simulink model "acDynModelGolfTenueClassique"  (R2019a)
settings: Solver=VariableStepAuto  StartTime=0.0  StopTime=10  RelTol=1e-3
values from neighbouring files (symbols this model uses):
  DEG2RAD = pi/180.    (= 0.0174532925199)    [mainProjetCADV_2a.m]    (also in utAcDynamicsFunction.m; utConstantAeroCoeff.m)
  dPHRTrim = trimVal(1)    [mainProjetCADV_2a.m]
  dthrIdle = 0.1    [mainProjetCADV_2a.m]
  km = trim.kmass(choix)    [utGetTrimPoint.m]
  ms = trim.mStat(choix)    [utGetTrimPoint.m]
  RAD2DEG = 180/pi    (= 57.2957795131)    [mainProjetCADV_2a.m]    (also in utAcDynamicsFunction.m)
  thetaTrim = trimVal(3)    [mainProjetCADV_2a.m]
  xTrim = zeros(TOTAL_SV, 1)    [mainProjetCADV_2a.m]
undefined symbols (not defined in the file or in its folder): aircraftChosen, Kd, Ki, Kp, state4den, state4num
settings Model: Creator=bourdiul  LastModifiedBy=ulyss

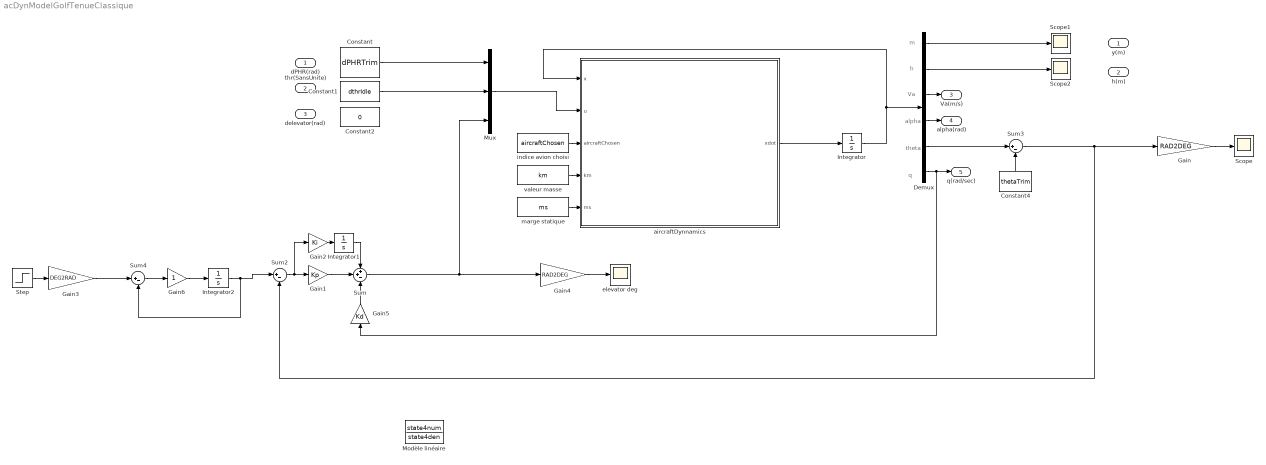
== system acDynModelGolfTenueClassique ==
  note: m
  note: h
  note: Va
  note: alpha
  note: theta
  note: q
  dPHR(rad) : Inport
  thr(SansUnite) : Inport  Port=2
  delevator(rad) : Inport  Port=3
  Constant : Constant  Value=dPHRTrim
  Constant1 : Constant  Value=dthrIdle
  Constant2 : Constant  Value=0
  Constant4 : Constant  Value=thetaTrim
  Demux : Demux  Outputs=6
  Gain : Gain  Gain=RAD2DEG
  Gain1 : Gain  Gain=Kp
  Gain2 : Gain  Gain=Ki
  Gain3 : Gain  Gain=DEG2RAD
  Gain4 : Gain  Gain=RAD2DEG
  Gain5 : Gain  Gain=Kd
  Gain6 : Gain
  Integrator : Integrator  InitialCondition=xTrim
  Integrator1 : Integrator
  Integrator2 : Integrator
  Modèle linéaire : TransferFcn  Numerator=state4num  Denominator=state4den
  Mux : Mux  Inputs=3
  Scope : Scope
  Scope1 : Scope
  Scope2 : Scope
  Step : Step  Time=0  After=5  SampleTime=0
  Sum : Sum  Inputs=++-
  Sum2 : Sum  Inputs=|+-
  Sum3 : Sum  Inputs=|+-
  Sum4 : Sum  Inputs=|+-
  aircraftDynnamics : MATLAB Function  TreatAsAtomicUnit=on
  elevator deg : Scope
  indice avion choisi : Constant  Value=aircraftChosen
  marge statique : Constant  Value=ms
  valeur masse : Constant  Value=km
  y(m) : Outport
  h(m) : Outport  Port=2
  Va(m/s) : Outport  Port=3
  alpha(rad) : Outport  Port=4
  q(rad/sec) : Outport  Port=5
  wires:
  marge statique/1 -> aircraftDynnamics/5(ms)
  Integrator/1 -> aircraftDynnamics/1(x), Demux/1
  Demux/6 -> Gain5/1, q(rad/sec)/1
  Mux/1 -> aircraftDynnamics/2(u)
  Demux/2 -> Scope2/1
  indice avion choisi/1 -> aircraftDynnamics/3(aircraftChosen)
  Demux/3 -> Va(m/s)/1
  valeur masse/1 -> aircraftDynnamics/4(km)
  aircraftDynnamics/1(xdot) -> Integrator/1
  Demux/4 -> alpha(rad)/1
  Constant1/1 -> Mux/2
  Constant/1 -> Mux/1
  Gain/1 -> Scope/1
  Demux/1 -> Scope1/1
  Gain5/1 -> Sum/3
  Step/1 -> Gain3/1
  Gain4/1 -> elevator deg/1
  Constant4/1 -> Sum3/2
  Gain1/1 -> Sum/2
  Integrator1/1 -> Sum/1
  Gain2/1 -> Integrator1/1
  Sum2/1 -> Gain2/1, Gain1/1
  Demux/5 -> Sum3/1
  Sum3/1 -> Gain/1, Sum2/2
  Sum/1 -> Mux/3, Gain4/1
  Integrator2/1 -> Sum2/1, Sum4/2
  Gain6/1 -> Integrator2/1
  Sum4/1 -> Gain6/1
  Gain3/1 -> Sum4/1

== matlab function acDynModelGolfTenueClassique/aircraftDynnamics ==
  data: x input; u input; xdot output; aircraftChosen input; km input; ms input
function xdot = aircraftDynamics(x,u, aircraftChosen,km,ms)
    TOTAL_SV = 6;
    xIn = zeros(TOTAL_SV,1);
    xIn = x;
    
	TOTAL_CMD = 3;
    uIn = zeros(TOTAL_CMD,1);
    uIn = u;
    
    xdot = utAcDynamicsFunction(xIn,uIn, aircraftChosen,km,ms);
end %aircraftDynamics
